simulink model "Trajektorie_TESTFILE"  (R2024a)
settings: Solver=VariableStepAuto  StartTime=0.0  StopTime=10.0  RelTol=1e-3
settings Model: Creator=apaul  LastModifiedBy=apaul

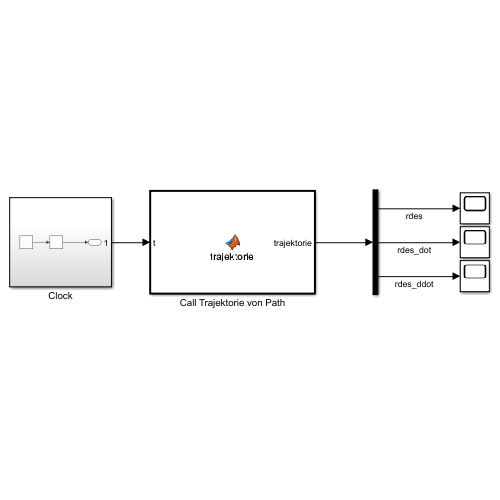
[thumbnail: Simulink's stored preview of the top-level diagram]
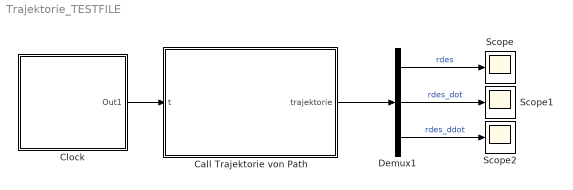
== system Trajektorie_TESTFILE ==
  Call Trajektorie von Path : MATLAB Function  TreatAsAtomicUnit=on
  Clock : Subsystem
  Demux1 : Demux  Outputs=3
  Scope : Scope
  Scope1 : Scope
  Scope2 : Scope
  wires:
  Clock/1(Out1) -> Call Trajektorie von Path/1(t)
  Demux1/2 -> Scope1/1  "rdes_dot"
  Call Trajektorie von Path/1(trajektorie) -> Demux1/1
  Demux1/1 -> Scope/1  "rdes"
  Demux1/3 -> Scope2/1  "rdes_ddot"

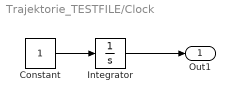
== system Trajektorie_TESTFILE/Clock ==
  Constant : Constant
  Integrator : Integrator
  Out1 : Outport
  wires:
  Constant/1 -> Integrator/1
  Integrator/1 -> Out1/1

== matlab function Trajektorie_TESTFILE/Call Trajektorie von Path ==
  data: trajektorie output; t input
function trajektorie = trajektorie(t)
%Trajektorie
%    TRAJEKTORIE = Trajektorie(T)

%    This function was generated by the Symbolic Math Toolbox version 24.1.
%    07-Jan-2025 10:14:32

t2 = t.^2;
t3 = t.^3;
t4 = t.*7.030674334031603e-2;
t5 = t.*5.130385555576637e-2;
t6 = t2.*2.565192777788319e-2;
t7 = t2.*3.515337167015802e-2;
trajektorie = [t3.*1.171779055671934e-2-t7;t3.*8.550642592627729e-3-t6-5.7e+1./2.5e+2;0.0;-t4+t7;-t5+t6;0.0;t4-7.030674334031603e-2;t5-5.130385555576637e-2;0.0];
end
